simulink model "soc_dvbs2_top_sw"  (R2025b)
settings: Solver=FixedStepDiscrete  StartTime=0.0  StopTime=inf  FixedStep=0.001  RelTol=1e-3  EnableMultiTasking=on
StartFcn:
  | warning('off', 'Simulink:Engine:ExtModeCannotDownloadParamBecauseNoHostToTarget');
StopFcn:
  | warning('on', 'Simulink:Engine:ExtModeCannotDownloadParamBecauseNoHostToTarget');
model workspace (MAT data in the model file):
  InterfaceBlocks = {'soc_dvbs2_proc/Processor Algorithm Periodic/ReadRegisters/Register Read'; 'soc_dvbs2_proc/Processor Algorithm Periodic/ReadRegisters/Register Read1'; 'soc_dvbs2_proc/Processor Algorithm Periodic/ReadRegisters/Register Read10'; 'soc_dvbs2_proc/Processor Algorithm Periodic/ReadRegisters/Register Read11'; 'soc_dvbs2_proc/Processor Algorithm Periodic/ReadRegisters/Register Read2'; 'soc_dvbs2_proc/Processor Algorithm Periodic/ReadRegisters/Register Read3'; 'soc_dvbs2_proc/Processor Algorithm Periodic/ReadRegisters/Register Read4'; 'soc_dvbs2_proc/Processor Algorithm Periodic/ReadRegisters/Register Read5'; 'soc_dvbs2_proc/Processor Algorithm Periodic/ReadRegisters/Register Read6'; 'soc_dvbs2_proc/Processor Algorithm Periodic/ReadRegisters/Register Read9'; 'soc_dvbs2_proc/Processor Algorithm Periodic/WriteRegisters/Register Write'; 'soc_dvbs2_proc/Processor Algorithm Periodic/WriteRegisters/Register Write1'; 'soc_dvbs2_proc/Processor Algorithm Periodic/WriteRegisters/Register Write10'; 'soc_dvbs2_proc/Processor Algorithm Periodic/WriteRegisters/Register Write2'; 'soc_dvbs2_proc/Processor Algorithm Periodic/WriteRegisters/Register Write3'; 'soc_dvbs2_proc/Processor Algorithm Periodic/WriteRegisters/Register Write4'; 'soc_dvbs2_proc/Processor Algorithm Periodic/WriteRegisters/Register Write6'; 'soc_dvbs2_proc/Processor Algorithm Periodic/WriteRegisters/Register Write8'}
undefined symbols (not defined in the file or in its folder): D1, P, RxFrameSize
libraries: prociodatalib x19, proctasklib x1
settings Model: SimulationMode=external  Creator=AEDemo  LastModifiedBy=KoayXianCong
settings SolverCC: AlgebraicLoopSolver=TrustRegion  PositivePriorityOrder=on  AutoInsertRateTranBlk=on
settings DataIOCC: SaveFormat=StructureWithTime  ReturnWorkspaceOutputs=off
settings OptimizationCC: DefaultParameterBehavior=Inlined  PassReuseOutputArgsAs=Individual arguments  ZeroExternalMemoryAtStartup=off  MaxStackSize=64  EfficientTunableParamExpr=on
settings DebuggingCC: InheritedTsInSrcMsg=none  IntegerOverflowMsg=none  ParameterTunabilityLossMsg=error  UnconnectedInputMsg=warning  UnconnectedOutputMsg=warning  UnconnectedLineMsg=warning  SubsystemReferenceDiagnosticForUnitTest=warning  ArithmeticOperatorsInVariantConditions=warning
settings HardwareCC: ProdBitPerLong=64.0  ProdLargestAtomicInteger=LongLong  ProdLargestAtomicFloat=Double  ProdLongLongMode=on  ProdHWDeviceType=ARM Compatible->ARM Cortex-A (64-bit)  HardwareBoardFeatureSet=SoCBlockset
settings ModelReferenceCC: EnableRefExpFcnMdlSchedulingChecks=on  ModelReferenceNumInstancesAllowed=Single
settings SFSimCC: SimUseLocalCustomCode=off
settings RTWCC: SystemTargetFile=ert.tlc  HardwareBoard=Xilinx Zynq UltraScale+ RFSoC ZCU111 Evaluation Kit  TLCOptions="-aInlineSetEventsForThisBaseRateFcn=TLC_FALSE -aSuppressMultiTaskScheduler=TLC_FALSE  -aRateBasedStepFcn=0"  TemplateMakefile=ert_default_tmf  GenerateReport=on  RTWUseLocalCustomCode=off  Toolchain=Linaro AArch64 Linux v6.3.1  IncludeHyperlinkInReport=on  LaunchReport=on  CodeExecutionProfiling=on  GenerateTraceInfo=on  GenerateTraceReport=on  GenerateTraceReportSl=on  GenerateTraceReportSf=on  GenerateTraceReportEml=on  GPUComputeCapability=3.5  DLArmComputeVersion=19.05  Description=Embedded Coder
settings CodeAppCC: ForceParamTrailComments=on  IgnoreCustomStorageClasses=off  OperatorAnnotations=on  SimulinkDataObjDesc=on  SFDataObjDesc=on  InsertBlockDesc=on
settings ERTTargetCC: InlinedParameterPlacement=Hierarchical  SupportVariableSizeSignals=on

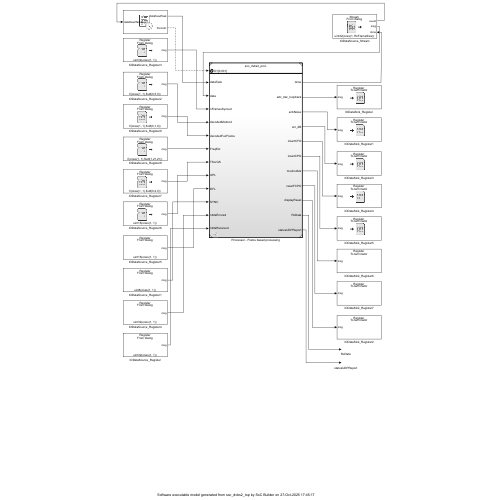
[thumbnail: Simulink's stored preview of the top-level diagram]
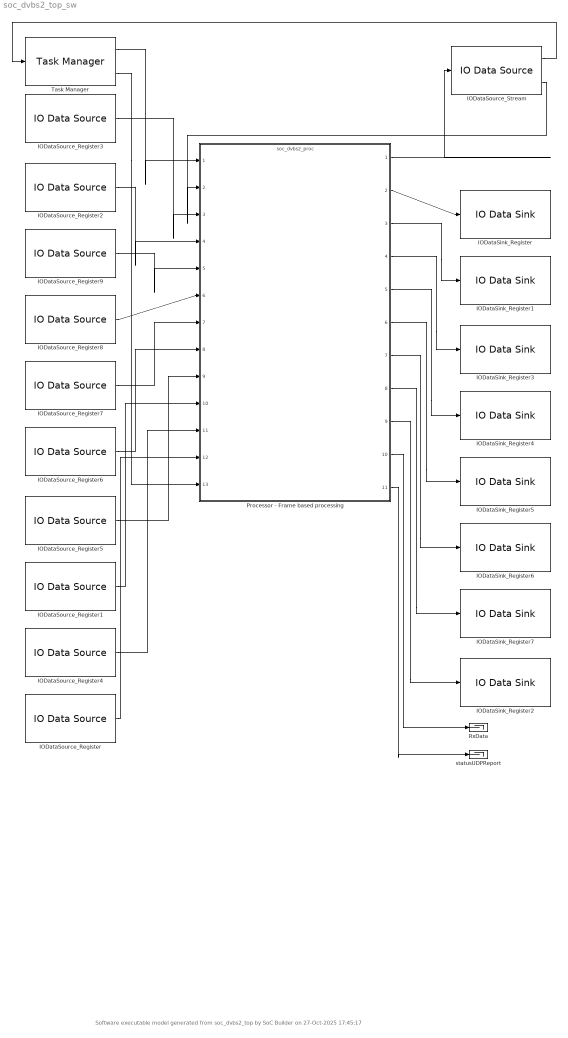
== system soc_dvbs2_top_sw ==
  note: Software executable model generated from soc_dvbs2_top by SoC Builder on 27-Oct-2025 17:45:17
  IODataSink_Register{,1..7} (8 alike) : prociodatalib/IO Data Sink  OutputSink=To terminator  DataTypeStr=uint32  Dimensions=1024  DeviceType=Register  EventDataPort=Data  QueueLength=8  SampleTime=-1  EnableDonePort=off
  IODataSource_Register : prociodatalib/IO Data Source  InputSource=From dialog  Value=uint32(ones(1, 1))  ObjectName=[]  DeviceType=Register  EventDataPort=Data  QueueLength=8  DataTypeStr=uint32  Dimensions=1024  ShowDonePort=off  SampleTime=inf  InternalSampleTime=inf
  IODataSource_Register1 : prociodatalib/IO Data Source  InputSource=From dialog  Value=uint8(ones(1, 1))  ObjectName=[]  DeviceType=Register  EventDataPort=Data  QueueLength=8  DataTypeStr=uint32  Dimensions=1024  ShowDonePort=off  SampleTime=inf  InternalSampleTime=inf
  IODataSource_Register2 : prociodatalib/IO Data Source  InputSource=From dialog  Value=fi(ones(1, 1),fixdt(0,5,0))  ObjectName=[]  DeviceType=Register  EventDataPort=Data  QueueLength=8  DataTypeStr=uint32  Dimensions=1024  ShowDonePort=off  SampleTime=inf  InternalSampleTime=inf
  IODataSource_Register3 : prociodatalib/IO Data Source  InputSource=From dialog  Value=uint32(ones(1, 1))  ObjectName=[]  DeviceType=Register  EventDataPort=Data  QueueLength=8  DataTypeStr=uint32  Dimensions=1024  ShowDonePort=off  SampleTime=inf  InternalSampleTime=inf
  IODataSource_Register4 : prociodatalib/IO Data Source  InputSource=From dialog  Value=uint32(ones(1, 1))  ObjectName=[]  DeviceType=Register  EventDataPort=Data  QueueLength=8  DataTypeStr=uint32  Dimensions=1024  ShowDonePort=off  SampleTime=inf  InternalSampleTime=inf
  IODataSource_Register5 : prociodatalib/IO Data Source  InputSource=From dialog  Value=uint16(ones(1, 1))  ObjectName=[]  DeviceType=Register  EventDataPort=Data  QueueLength=8  DataTypeStr=uint32  Dimensions=1024  ShowDonePort=off  SampleTime=inf  InternalSampleTime=inf
  IODataSource_Register6 : prociodatalib/IO Data Source  InputSource=From dialog  Value=uint16(ones(1, 1))  ObjectName=[]  DeviceType=Register  EventDataPort=Data  QueueLength=8  DataTypeStr=uint32  Dimensions=1024  ShowDonePort=off  SampleTime=inf  InternalSampleTime=inf
  IODataSource_Register7 : prociodatalib/IO Data Source  InputSource=From dialog  Value=fi(ones(1, 1),fixdt(0,2,0))  ObjectName=[]  DeviceType=Register  EventDataPort=Data  QueueLength=8  DataTypeStr=uint32  Dimensions=1024  ShowDonePort=off  SampleTime=inf  InternalSampleTime=inf
  IODataSource_Register8 : prociodatalib/IO Data Source  InputSource=From dialog  Value=fi(ones(1, 1),fixdt(1,21,21))  ObjectName=[]  DeviceType=Register  EventDataPort=Data  QueueLength=8  DataTypeStr=uint32  Dimensions=1024  ShowDonePort=off  SampleTime=inf  InternalSampleTime=inf
  IODataSource_Register9 : prociodatalib/IO Data Source  InputSource=From dialog  Value=fi(ones(1, 1),fixdt(0,1,0))  ObjectName=[]  DeviceType=Register  EventDataPort=Data  QueueLength=8  DataTypeStr=uint32  Dimensions=1024  ShowDonePort=off  SampleTime=inf  InternalSampleTime=inf
  IODataSource_Stream : prociodatalib/IO Data Source  InputSource=From dialog  Value=uint32(ones(1, RxFrameSize))  ObjectName=[]  DeviceType=Stream  EventDataPort=Data and Event  QueueLength=4  DataTypeStr=uint32  Dimensions=1024  ShowDonePort=on  SampleTime=inf  InternalSampleTime=inf
  Processor - Frame based processing : ModelReference  LoadFcn=|  ModelNameDialog=soc_dvbs2_proc.slx  SimulationMode=Normal  ScheduleRates=on  CachedPortDiscreteRates=[0.001]  ModelEventPortInfo=P:D1[0.001][0][0]  ModelReferenceVersion=11.0
      | load_system('soc_dvbs2_proc');
      | 
      | set_param('soc_dvbs2_proc/Processor Algorithm Periodic/ReadRegisters/Register Read', 'DeviceName', '/dev/mwdvbs2_ip0');
      | set_param('soc_dvbs2_proc/Processor Algorithm Periodic/ReadRegisters/Register Read', 'OffsetAddress', 'hex2dec(''0124'')');
      | set_param('soc_dvbs2_proc/Processor Algorithm Periodic/ReadRegisters/Register Read1', 'DeviceName', '/dev/mwdvbs2_ip0');
      | set_param('soc_dvbs2_proc/Processor Algorithm Periodic/ReadRegisters/Register Read1', 'OffsetAddress', 'hex2dec(''011C'')');
      | set_param('soc_dvbs2_proc/Processor Algorithm Periodic/ReadRegisters/Register Read10', 'DeviceName', '/dev/mwdvbs2_ip0');
      | set_param('soc_dvbs2_proc/Processor Algorithm Periodic/ReadRegisters/Register Read10', 'OffsetAddress', 'hex2dec(''0104'')');
      | set_param('soc_dvbs2_proc/Processor Algorithm Periodic/ReadRegisters/Register Read11', 'DeviceName', '/dev/mwdvbs2_ip0');
      | set_param('soc_dvbs2_proc/Processor Algorithm Periodic/ReadRegisters/Register Read11', 'OffsetAddress', 'hex2dec(''0100'')');
      | set_param('soc_dvbs2_proc/Processor Algorithm Periodic/ReadRegisters/Register Read2', 'DeviceName', '/dev/mwdvbs2_ip0');
      | set_param('soc_dvbs2_proc/Processor Algorithm Periodic/ReadRegisters/Register Read2', 'OffsetAddress', 'hex2dec(''0120'')');
      | set_param('soc_dvbs2_proc/Processor Algorithm Periodic/ReadRegisters/Register Read3', 'DeviceName', '/dev/mwdvbs2_ip0');
      | set_param('soc_dvbs2_proc/Processor Algorithm Periodic/ReadRegisters/Register Read3', 'OffsetAddress', 'hex2dec(''0118'')');
      | set_param('soc_dvbs2_proc/Processor Algorithm Periodic/ReadRegisters/Register Read4', 'DeviceName', '/dev/mwdvbs2_ip0');
      | set_param('soc_dvbs2_proc/Processor Algorithm Periodic/ReadRegisters/Register Read4', 'OffsetAddress', 'hex2dec(''0114'')');
      | set_param('soc_dvbs2_proc/Processor Algorithm Periodic/ReadRegisters/Register Read5', 'DeviceName', '/dev/mwdvbs2_ip0');
      | set_param('soc_dvbs2_proc/Processor Algorithm Periodic/ReadRegisters/Register Read5', 'OffsetAddress', 'hex2dec(''0110'')');
      | set_param('soc_dvbs2_proc/Processor Algorithm Periodic/ReadRegisters/Register Read6', 'DeviceName', '/dev/mwdvbs2_ip0');
      | set_param('soc_dvbs2_proc/Processor Algorithm Periodic/ReadRegisters/Register Read6', 'OffsetAddress', 'hex2dec(''010C'')');
      | set_param('soc_dvbs2_proc/Processor Algorithm Periodic/ReadRegisters/Register Read9', 'DeviceName', '/dev/mwdvbs2_ip0');
      | set_param('soc_dvbs2_proc/Processor Algorithm Periodic/ReadRegisters/Register Read9', 'OffsetAddress', 'hex2dec(''0108'')');
      | set_param('soc_dvbs2_proc/Processor Algorithm Periodic/WriteRegisters/Register Write', 'DeviceName', '/dev/mwdvbs2_ip0');
      | set_param('soc_dvbs2_proc/Processor Algorithm Periodic/WriteRegisters/Register Write', 'OffsetAddress', 'hex2dec(''0128'')');
      | set_param('soc_dvbs2_proc/Processor Algorithm Periodic/WriteRegisters/Register Write1', 'DeviceName', '/dev/mwdvbs2_ip0');
      | set_param('soc_dvbs2_proc/Processor Algorithm Periodic/WriteRegisters/Register Write1', 'OffsetAddress', 'hex2dec(''012C'')');
      | set_param('soc_dvbs2_proc/Processor Algorithm Periodic/WriteRegisters/Register Write10', 'DeviceName', '/dev/mwdvbs2_ip0');
      | set_param('soc_dvbs2_proc/Processor Algorithm Periodic/WriteRegisters/Register Write10', 'OffsetAddress', 'hex2dec(''0144'')');
      | set_param('soc_dvbs2_proc/Processor Algorithm Periodic/WriteRegisters/Register Write2', 'DeviceName', '/dev/mwdvbs2_ip0');
      | set_param('soc_dvbs2_proc/Processor Algorithm Periodic/WriteRegisters/Register Write2', 'OffsetAddress', 'hex2dec(''0130'')');
      | set_param('soc_dvbs2_proc/Processor Algorithm Periodic/WriteRegisters/Register Write3', 'DeviceName', '/dev/mwdvbs2_ip0');
      | set_param('soc_dvbs2_proc/Processor Algorithm Periodic/WriteRegisters/Register Write3', 'OffsetAddress', 'hex2dec(''0134'')');
      | set_param('soc_dvbs2_proc/Processor Algorithm Periodic/WriteRegisters/Register Write4', 'DeviceName', '/dev/mwdvbs2_ip0');
      | set_param('soc_dvbs2_proc/Processor Algorithm Periodic/WriteRegisters/Register Write4', 'OffsetAddress', 'hex2dec(''0138'')');
      | set_param('soc_dvbs2_proc/Processor Algorithm Periodic/WriteRegisters/Register Write6', 'DeviceName', '/dev/mwdvbs2_ip0');
      | set_param('soc_dvbs2_proc/Processor Algorithm Periodic/WriteRegisters/Register Write6', 'OffsetAddress', 'hex2dec(''013C'')');
      | set_param('soc_dvbs2_proc/Processor Algorithm Periodic/WriteRegisters/Register Write8', 'DeviceName', '/dev/mwdvbs2_ip0');
      | set_param('soc_dvbs2_proc/Processor Algorithm Periodic/WriteRegisters/Register Write8', 'OffsetAddress', 'hex2dec(''0140'')');
      | set_param('soc_dvbs2_proc/Read Event/Stream Read', 'DeviceName', 'mwdvbs2_ip0:s2mm0');
      | set_param('soc_dvbs2_proc', 'Dirty','off');
  RxData : Terminator
  Task Manager : proctasklib/Task Manager  AllTaskData="[{\"taskName\":\"dataReadTask\",\"taskType\":\"Event-driven\",\"taskEvent\":\"dataReadTaskEvent\",\"taskPeriod\":\"0.1\",\"taskPriority\":\"50\",\"coreSelection\":\"Specified core\",\"coreNum\":\"0\",\"dropOverranTasks\":false,\"playbackRecorded\":false,\"diagnosticsFile\":\"\",\"taskDurationSource\":\"Dialog\",\"taskDuration\":1E-6,\"taskDurationDeviation\":0,\"logExecutionData\":true,\"logDroppedTasks\":false,\"version\":\"2.6\",\"taskDurationData\":{\"percent\":[\"100\"],\"mean\":[\"1e-06\"],\"dev\":[\"0\"],\"min\":[\"1e-06\"],\"max\":[\"1e-06\"]},\"taskEventSource\":\"IODataSource_Stream\",\"taskEventSourceAssignmentType\":\"ManuallyAssigned\",\"taskEventSourceType\":\"Stream\",\"taskEventGroup\":\"Unspecified\",\"taskEventInterrupt\":\"Unspecified\",\"taskEventOrder\":1,\"taskDisablePremption\":false,\"taskClearInterruptFlagsAtEndOfEvent\":false},{\"taskName\":\"Periodic\",\"taskType\":\"Timer-driven\",\"taskEvent\":\"PeriodicEvent\",\"taskPeriod\":\"1e-3\",\"taskPriority\":\"51\",\"coreSelection\":\"Specified core\",\"coreNum\":\"0\",\"dropOverranTasks\":false,\"playbackRecorded\":false,\"diagnosticsFile\":\"\",\"taskDurationSource\":\"Dialog\",\"taskDuration\":1E-6,\"taskDurationDeviation\":0,\"logExecutionData\":true,\"logDroppedTasks\":false,\"version\":\"2.6\",\"taskDurationData\":{\"percent\":[\"100\"],\"mean\":[\"1e-06\"],\"dev\":[\"0\"],\"min\":[\"1e-06\"],\"max\":[\"1e-06\"]},\"taskEventSource\":\"Internal\",\"taskEventSourceAssignmentType\":\"AutoAssigned\",\"taskEventSourceType\":\"Unspecified\",\"taskEventGroup\":\"Unspecified\",\"taskEventInterrupt\":\"Unspecified\",\"taskEventOrder\":1,\"taskDisablePremption\":false,\"taskClearInterruptFlagsAtEndOfEvent\":false}]"  EnableTaskSimulation=on  StreamToSDI=on  WriteToFile=off  OverwriteFile=off  SupportEventPorts=on  UseScheduleEditor=off  CustomizationInfo=''
  statusUDPReport : Terminator
  wires:
  Task Manager/2 -> Processor - Frame based processing/13
  Processor - Frame based processing/6 -> IODataSink_Register5/1
  Task Manager/1 -> Processor - Frame based processing/1
  IODataSource_Register3/1 -> Processor - Frame based processing/3
  IODataSource_Register9/1 -> Processor - Frame based processing/5
  IODataSource_Register2/1 -> Processor - Frame based processing/4
  IODataSource_Register8/1 -> Processor - Frame based processing/6
  Processor - Frame based processing/2 -> IODataSink_Register/1
  IODataSource_Register7/1 -> Processor - Frame based processing/7
  IODataSource_Register6/1 -> Processor - Frame based processing/8
  IODataSource_Register5/1 -> Processor - Frame based processing/9
  IODataSource_Register1/1 -> Processor - Frame based processing/10
  IODataSource_Register4/1 -> Processor - Frame based processing/11
  IODataSource_Register/1 -> Processor - Frame based processing/12
  Processor - Frame based processing/1 -> IODataSource_Stream/1
  Processor - Frame based processing/3 -> IODataSink_Register1/1
  Processor - Frame based processing/4 -> IODataSink_Register3/1
  Processor - Frame based processing/5 -> IODataSink_Register4/1
  Processor - Frame based processing/7 -> IODataSink_Register6/1
  Processor - Frame based processing/8 -> IODataSink_Register7/1
  Processor - Frame based processing/9 -> IODataSink_Register2/1
  Processor - Frame based processing/10 -> RxData/1
  Processor - Frame based processing/11 -> statusUDPReport/1
  IODataSource_Stream/1 -> Task Manager/1
  IODataSource_Stream/2 -> Processor - Frame based processing/2
